simulink model "controllerCh6"  (R2014a)
settings: configuration reference "globalConfig" (kept outside this file)
undefined symbols (not defined in the file): digital_range, direction_range, duty_range, gcbh, normalized_range, rmidispblock, Ts, uint_range_10bit
settings Model: Creator=jrivitus  LastModifiedBy=scastro

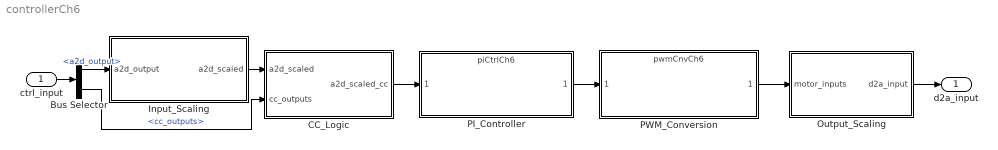
== system controllerCh6 ==
  ctrl_input : Inport  OutDataTypeStr=Bus: ctrl_input_bus  PortDimensions=1  SampleTime=Ts
  Bus Selector : BusSelector  OutputSignals=a2d_output,cc_outputs
  CC_Logic : Subsystem  TreatAsAtomicUnit=on
  Input_Scaling : Subsystem  RequirementInfo={'other' 'throttleReqsCh6.doc' '@inp_scl_1' 'true' 'Scaled data must be responsive to full range of input data.' '' ; 'other' 'throttleReqsCh6.doc' '@inp_scl_2' 'true' 'Output range for each signal must be normalized.' '' } %GIDa_d12db97f_5d84_4f01_aa73_1a00163fa707  TreatAsAtomicUnit=on
  Output_Scaling : Subsystem  RequirementInfo={'other' 'throttleReqsCh6.doc' '@out_scl_1' 'true' 'Scaled data must be responsive to full range of input data.' '' ; 'other' 'throttleReqsCh6.doc' '@out_scl_2' 'true' 'Output data must be scaled for direct input to driver software' '' } %GIDa_040f54b5_feae_4999_b3ff_f49e3529df7e  TreatAsAtomicUnit=on
  PI_Controller : ModelReference  ModelNameDialog=piCtrlCh6  SimulationMode=Normal  ModelReferenceVersion=1.123  CopyOfModelName=piCtrlCh6  DefaultDataLogging=off
  PWM_Conversion : ModelReference  ModelNameDialog=pwmCnvCh6  SimulationMode=Normal  ModelReferenceVersion=1.124  CopyOfModelName=pwmCnvCh6  DefaultDataLogging=off
  d2a_input : Outport  OutDataTypeStr=Bus: d2a_input_bus  SampleTime=Ts
  wires:
  Output_Scaling/1(d2a_input) -> d2a_input/1
  PWM_Conversion/1 -> Output_Scaling/1(motor_inputs)
  PI_Controller/1 -> PWM_Conversion/1
  Input_Scaling/1(a2d_scaled) -> CC_Logic/1(a2d_scaled)
  Bus Selector/1 -> Input_Scaling/1(a2d_output)  "<a2d_output>"
  ctrl_input/1 -> Bus Selector/1
  CC_Logic/1(a2d_scaled_cc) -> PI_Controller/1
  Bus Selector/2 -> CC_Logic/2(cc_outputs)  "<cc_outputs>"

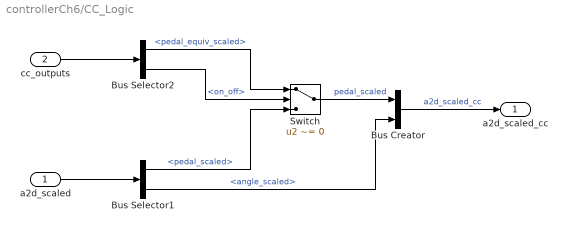
== system controllerCh6/CC_Logic ==
  a2d_scaled : Inport  OutDataTypeStr=Bus: a2d_scaled_bus  SampleTime=Ts
  cc_outputs : Inport  Port=2  OutDataTypeStr=Bus: cc_outputs_bus  SampleTime=Ts
  Bus Creator : BusCreator  Inputs=2
  Bus Selector1 : BusSelector  OutputSignals=pedal_scaled,angle_scaled
  Bus Selector2 : BusSelector  OutputSignals=pedal_equiv_scaled,on_off
  Switch : Switch  Criteria=u2 ~= 0
      settings: AttributesFormatString="Criteria for passing\\nsignal 1:  %<Criteria>"
  a2d_scaled_cc : Outport  OutDataTypeStr=Bus: a2d_scaled_bus  SampleTime=[0.01,0]
  wires:
  Bus Selector2/2 -> Switch/2  "<on_off>"
  Bus Selector2/1 -> Switch/1  "<pedal_equiv_scaled>"
  Bus Selector1/1 -> Switch/3  "<pedal_scaled>"
  Switch/1 -> Bus Creator/1  "pedal_scaled"
  cc_outputs/1 -> Bus Selector2/1
  Bus Creator/1 -> a2d_scaled_cc/1  "a2d_scaled_cc"
  Bus Selector1/2 -> Bus Creator/2  "<angle_scaled>"
  a2d_scaled/1 -> Bus Selector1/1

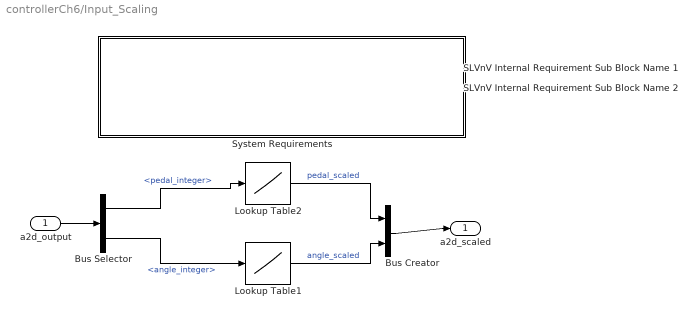
== system controllerCh6/Input_Scaling ==
  a2d_output : Inport  OutDataTypeStr=Bus: a2d_output_bus  PortDimensions=1  SampleTime=Ts
  Bus Creator : BusCreator  Inputs=2  OutDataTypeStr=Bus: a2d_scaled_bus
  Bus Selector : BusSelector  OutputSignals=pedal_integer,angle_integer
  Lookup Table1 : Lookup_n-D  NumberOfTableDimensions=1  BreakpointsForDimension1=uint_range_10bit  Table=normalized_range  ExtrapMethod=Clip  OutDataTypeStr=double  InputSameDT=on
      settings: AttributesFormatString=Output data type: %<OutDataTypeStr>
  Lookup Table2 : Lookup_n-D  NumberOfTableDimensions=1  BreakpointsForDimension1=uint_range_10bit  Table=normalized_range  ExtrapMethod=Clip  OutDataTypeStr=double  InputSameDT=on
      settings: AttributesFormatString=Output data type: %<OutDataTypeStr>
  SLVnV Internal Requirement Sub Block Name 1 : Subsystem  mask(System Requirement Item){label=0, index=1}
      mask init:
      | label = rmidispblock('label',index);
      settings: CopyFcn=rmidispblock('copyReq',gcbh)  DeleteFcn=rmidispblock('deleteReq',gcbh);  OpenFcn=rmidispblock('openReq',gcbh)  MoveFcn=rmidispblock('move',gcbh);
      mask Display: text(0,0,label,'horizontalAlignment','left','verticalAlignment','bottom')
  SLVnV Internal Requirement Sub Block Name 2 : Subsystem  mask(System Requirement Item){label=0, index=2}
      mask init:
      | label = rmidispblock('label',index);
      settings: CopyFcn=rmidispblock('copyReq',gcbh)  DeleteFcn=rmidispblock('deleteReq',gcbh);  OpenFcn=rmidispblock('openReq',gcbh)  MoveFcn=rmidispblock('move',gcbh);
      mask Display: text(0,0,label,'horizontalAlignment','left','verticalAlignment','bottom')
  System Requirements : Subsystem  LoadFcn=rmidispblock('load',gcbh)  mask(System Requirements){id=SystemReq, title=System Requirements}
      mask prompts: title "Block Title"
      mask help: Lists the requirements for the current model.
      mask init:
      | id = 'SystemReq';
      | [w,h] = rmidispblock('display',gcbh);
      settings: CopyFcn=rmidispblock('create',gcbh)  DeleteFcn=rmidispblock('delete',gcbh)  ModelCloseFcn=rmidispblock('close',gcbh)  PreSaveFcn=rmidispblock('close',gcbh)  PostSaveFcn=rmidispblock('open',gcbh)  OpenFcn=rmidispblock('open',gcbh)  MoveFcn=rmidispblock('move',gcbh)
      mask Help: helpview(fullfile(docroot,'toolbox','slvnv','slvnv.map'),'systemrequirements')
      mask Display: text(363/2,97-4,rmidispblock('title',gcbh),'horizontalAlignment','center','verticalAlignment','top')
  a2d_scaled : Outport  OutDataTypeStr=Bus: a2d_scaled_bus  SampleTime=Ts
  wires:
  Bus Creator/1 -> a2d_scaled/1
  a2d_output/1 -> Bus Selector/1
  Lookup Table1/1 -> Bus Creator/2  "angle_scaled"
  Bus Selector/2 -> Lookup Table1/1  "<angle_integer>"
  Lookup Table2/1 -> Bus Creator/1  "pedal_scaled"
  Bus Selector/1 -> Lookup Table2/1  "<pedal_integer>"

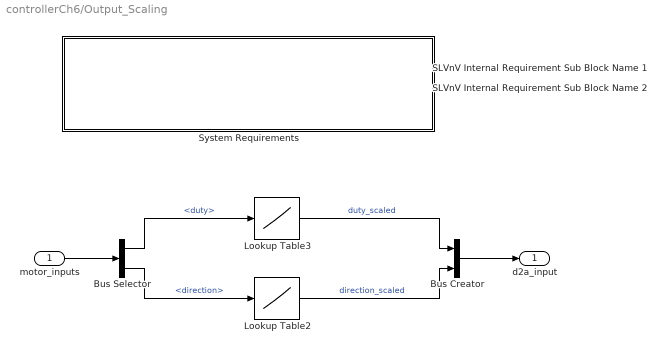
== system controllerCh6/Output_Scaling ==
  motor_inputs : Inport  OutDataTypeStr=Bus: motor_inputs_bus  PortDimensions=1  SampleTime=Ts
  Bus Creator : BusCreator  Inputs=2  OutDataTypeStr=Bus: d2a_input_bus
  Bus Selector : BusSelector  OutputSignals=duty,direction
  Lookup Table2 : Lookup_n-D  NumberOfTableDimensions=1  BreakpointsForDimension1=direction_range  Table=digital_range  ExtrapMethod=Clip  OutDataTypeStr=uint16  InputSameDT=on
      settings: AttributesFormatString=Output data type: %<OutDataTypeStr>
  Lookup Table3 : Lookup_n-D  NumberOfTableDimensions=1  BreakpointsForDimension1=duty_range  Table=uint_range_10bit  ExtrapMethod=Clip  OutDataTypeStr=uint16  InputSameDT=on
      settings: AttributesFormatString=Output data type: %<OutDataTypeStr>
  SLVnV Internal Requirement Sub Block Name 1 : Subsystem  mask(System Requirement Item){label=0, index=1}
      mask init:
      | label = rmidispblock('label',index);
      settings: CopyFcn=rmidispblock('copyReq',gcbh)  DeleteFcn=rmidispblock('deleteReq',gcbh);  OpenFcn=rmidispblock('openReq',gcbh)  MoveFcn=rmidispblock('move',gcbh);
      mask Display: text(0,0,label,'horizontalAlignment','left','verticalAlignment','bottom')
  SLVnV Internal Requirement Sub Block Name 2 : Subsystem  mask(System Requirement Item){label=0, index=2}
      mask init:
      | label = rmidispblock('label',index);
      settings: CopyFcn=rmidispblock('copyReq',gcbh)  DeleteFcn=rmidispblock('deleteReq',gcbh);  OpenFcn=rmidispblock('openReq',gcbh)  MoveFcn=rmidispblock('move',gcbh);
      mask Display: text(0,0,label,'horizontalAlignment','left','verticalAlignment','bottom')
  System Requirements : Subsystem  LoadFcn=rmidispblock('load',gcbh)  mask(System Requirements){id=SystemReq, title=System Requirements}
      mask prompts: title "Block Title"
      mask help: Lists the requirements for the current model.
      mask init:
      | id = 'SystemReq';
      | [w,h] = rmidispblock('display',gcbh);
      settings: CopyFcn=rmidispblock('create',gcbh)  DeleteFcn=rmidispblock('delete',gcbh)  ModelCloseFcn=rmidispblock('close',gcbh)  PreSaveFcn=rmidispblock('close',gcbh)  PostSaveFcn=rmidispblock('open',gcbh)  OpenFcn=rmidispblock('open',gcbh)  MoveFcn=rmidispblock('move',gcbh)
      mask Help: helpview(fullfile(docroot,'toolbox','slvnv','slvnv.map'),'systemrequirements')
      mask Display: text(368/2,91-4,rmidispblock('title',gcbh),'horizontalAlignment','center','verticalAlignment','top')
  d2a_input : Outport  OutDataTypeStr=Bus: d2a_input_bus  SampleTime=Ts
  wires:
  motor_inputs/1 -> Bus Selector/1
  Bus Creator/1 -> d2a_input/1
  Lookup Table2/1 -> Bus Creator/2  "direction_scaled"
  Bus Selector/2 -> Lookup Table2/1  "<direction>"
  Bus Selector/1 -> Lookup Table3/1  "<duty>"
  Lookup Table3/1 -> Bus Creator/1  "duty_scaled"

== system controllerCh6/Input_Scaling/SLVnV Internal Requirement Sub Block Name 1 ==

== system controllerCh6/Input_Scaling/SLVnV Internal Requirement Sub Block Name 2 ==

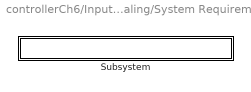
== system controllerCh6/Input_Scaling/System Requirements ==
  Subsystem : Subsystem  mask{label=0, index=1}
      mask init:
      | label = rmidispblock('label',index);
      settings: OpenFcn=rmidispblock('openReq',gcbh);
      mask Display: text(0,0,label,'horizontalAlignment','left','verticalAlignment','bottom')

== system controllerCh6/Output_Scaling/SLVnV Internal Requirement Sub Block Name 1 ==

== system controllerCh6/Output_Scaling/SLVnV Internal Requirement Sub Block Name 2 ==

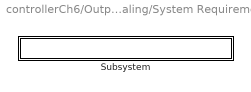
== system controllerCh6/Output_Scaling/System Requirements ==
  Subsystem : Subsystem  mask{label=0, index=1}
      mask init:
      | label = rmidispblock('label',index);
      settings: OpenFcn=rmidispblock('openReq',gcbh);
      mask Display: text(0,0,label,'horizontalAlignment','left','verticalAlignment','bottom')

== system controllerCh6/Input_Scaling/System Requirements/Subsystem ==

== system controllerCh6/Output_Scaling/System Requirements/Subsystem ==
